simulink model "Offline_Preprocessing_ECGandSCG3D"  (R2019a)
settings: Solver=FixedStepDiscrete  StartTime=0.0  StopTime=param_sim_time  FixedStep=1/fs  MaxStep=1/fs  RelTol=1e-3
undefined symbols (not defined in the file): fdesignblkfcn, fs, gcbh
(part 1 of 3)
settings Model: PacingRate=100  Creator=rcord  LastModifiedBy=rcord
settings SolverCC: ZeroCrossControl=DisableAll
settings DataIOCC: ExternalInput=[t, signals.ecg.input, signals.scg.input_xyz]  LoadExternalInput=on  SignalLogging=off  DSMLogging=off  SaveTime=off  ReturnWorkspaceOutputs=off  TimeSaveName=t_preprocessing  OutputSaveName=out_preprocessing  LoggingIntervals=[-inf,inf]

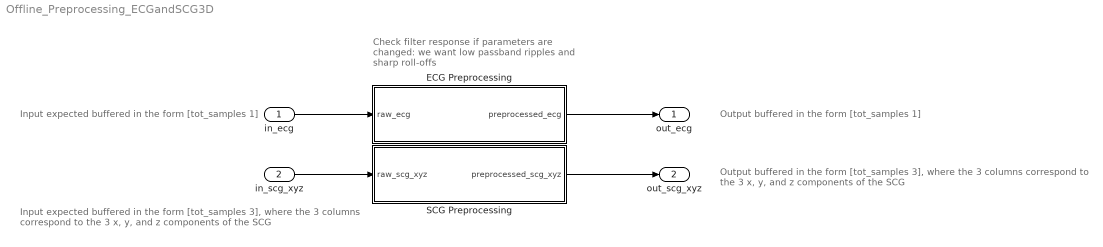
== system Offline_Preprocessing_ECGandSCG3D ==
  note: Input expected buffered in the form [tot_samples 3],
      | where the 3 columns correspond to the 3 x, y, and z components of the SCG
  note: Input expected buffered in the form [tot_samples 1]
  note: Check filter response if parameters are changed:
      | we want low passband ripples and sharp roll-offs
  note: Output buffered in the form [tot_samples 1]
  note: Output buffered in the form [tot_samples 3],
      | where the 3 columns correspond to the 3 x, y, and z components of the SCG
  in_ecg : Inport  SampleTime=1/fs
  in_scg_xyz : Inport  Port=2  SampleTime=1/fs
  ECG Preprocessing : Subsystem  mask{param_ecg_gain_mv=1000, param_ecg_fc_lo=2.05, param_ecg_fc_hi=36, param_ecg_trans_bw=2}
      mask prompts: param_ecg_gain_mv "mV Conversion Gain"; param_ecg_fc_lo "Low Passband Frequency Corner (Hz)"; param_ecg_fc_hi "High Passband Frequency Corner (Hz)"; param_ecg_trans_bw "Transition Bandwidth (Hz)"
      mask init:
      | assignin('base','param_ecg_gain_mv',param_ecg_gain_mv)
      | assignin('base','param_ecg_fc_lo',param_ecg_fc_lo)
      | assignin('base','param_ecg_fc_hi',param_ecg_fc_hi)
      | assignin('base','param_ecg_trans_bw',param_ecg_trans_bw)
      mask DialogControl DescGroupVar Prompt: ECG Preprocessing
      mask DialogControl DescTextVar Prompt: Preprocessing stage of the ECG. This involves conversion from V to mV and a filtfilt operation (i.e. a zero-phase FIR filtering) specified by the passband cornerns and transition bandwidth.
  SCG Preprocessing : Subsystem  mask{param_scg_gain_mg=3333, param_scg_fc_lo=7.5, param_scg_fc_hi=40, param_scg_trans_bw=2.5}
      mask prompts: param_scg_gain_mg "V to mg Conversion Gain"; param_scg_fc_lo "Low Passband Frequency Corner (Hz)"; param_scg_fc_hi "High Passband Frequency Corner (Hz)"; param_scg_trans_bw "Transition bandwidth"
      mask init:
      | assignin('base','param_scg_gain_mg',param_scg_gain_mg)
      | assignin('base','param_scg_fc_lo',param_scg_fc_lo)
      | assignin('base','param_scg_fc_hi',param_scg_fc_hi)
      | assignin('base','param_scg_trans_bw',param_scg_trans_bw)
      mask DialogControl DescGroupVar Prompt: SCG Preprocessing
      mask DialogControl DescTextVar Prompt: The SCG (x, y, and z) preprocessing block. This involves a V to mg conversion (determined by the transducer sensitivity) and a filtfilt operation. This filtfilt operation consists of a zero-phase FIR front-back filtering that is identical for each of the three cartesian acceleration components and is specified by the passband frequency corners and the transition bandwidth.
  out_ecg : Outport
  out_scg_xyz : Outport  Port=2
  wires:
  SCG Preprocessing/1(preprocessed_scg_xyz) -> out_scg_xyz/1
  ECG Preprocessing/1(preprocessed_ecg) -> out_ecg/1
  in_ecg/1 -> ECG Preprocessing/1(raw_ecg)
  in_scg_xyz/1 -> SCG Preprocessing/1(raw_scg_xyz)

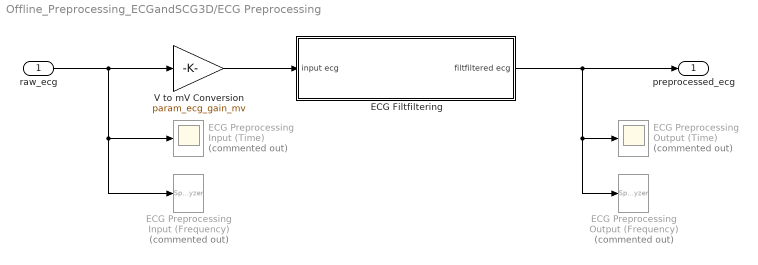
== system Offline_Preprocessing_ECGandSCG3D/ECG Preprocessing ==
  raw_ecg : Inport
  ECG Filtfiltering : Subsystem
  ECG Preprocessing Input (Frequency) : SpectrumAnalyzer  Commented=on
  ECG Preprocessing Input (Time) : Scope  Commented=on
  ECG Preprocessing Output (Frequency) : SpectrumAnalyzer  Commented=on
  ECG Preprocessing Output (Time) : Scope  Commented=on
  V to mV Conversion : Gain  Gain=param_ecg_gain_mv
  preprocessed_ecg : Outport
  wires:
  ECG Filtfiltering/1(filtfiltered ecg) -> preprocessed_ecg/1, ECG Preprocessing Output (Frequency)/1, ECG Preprocessing Output (Time)/1
  raw_ecg/1 -> V to mV Conversion/1, ECG Preprocessing Input (Frequency)/1, ECG Preprocessing Input (Time)/1
  V to mV Conversion/1 -> ECG Filtfiltering/1(input ecg)

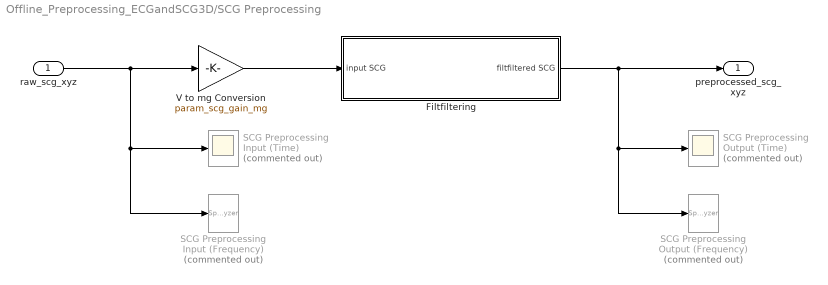
== system Offline_Preprocessing_ECGandSCG3D/SCG Preprocessing ==
  raw_scg_xyz : Inport
  Filtfiltering : Subsystem
  SCG Preprocessing Input (Frequency) : SpectrumAnalyzer  Commented=on
  SCG Preprocessing Input (Time) : Scope  Commented=on
  SCG Preprocessing Output (Frequency) : SpectrumAnalyzer  Commented=on
  SCG Preprocessing Output (Time) : Scope  Commented=on
  V to mg Conversion : Gain  Gain=param_scg_gain_mg
  preprocessed_scg_xyz : Outport
  wires:
  V to mg Conversion/1 -> Filtfiltering/1(" input SCG")
  Filtfiltering/1(filtfiltered SCG) -> preprocessed_scg_xyz/1, SCG Preprocessing Output (Frequency)/1, SCG Preprocessing Output (Time)/1
  raw_scg_xyz/1 -> V to mg Conversion/1, SCG Preprocessing Input (Frequency)/1, SCG Preprocessing Input (Time)/1

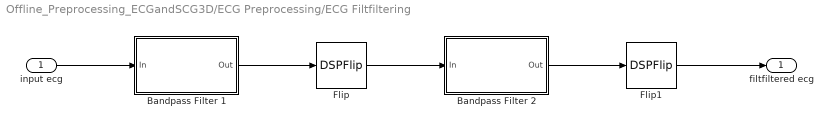
== system Offline_Preprocessing_ECGandSCG3D/ECG Preprocessing/ECG Filtfiltering ==
  input ecg : Inport
  Bandpass Filter 1 : Subsystem  DialogController=fdesignblkfcn  InitFcn=fdesignblkfcn(gcbh, {'InitFcn'});  mask(Bandpass Filter){}
      mask help: Design a bandpass filter
      settings: CopyFcn=fdesignblkfcn(gcbh, {'CopyFcn'});
      mask Help: helpview(mapfilelocation('dsp'), 'dspbandpassfilter');
      mask Display: disp('Bandpass');
  Bandpass Filter 2 : Subsystem  DialogController=fdesignblkfcn  InitFcn=fdesignblkfcn(gcbh, {'InitFcn'});  mask(Bandpass Filter){}
      mask help: Design a bandpass filter
      settings: CopyFcn=fdesignblkfcn(gcbh, {'CopyFcn'});
      mask Help: helpview(mapfilelocation('dsp'), 'dspbandpassfilter');
      mask Display: disp('Bandpass');
  Flip : DSPFlip
  Flip1 : DSPFlip
  filtfiltered ecg : Outport
  wires:
  Flip/1 -> Bandpass Filter 2/1(In)
  input ecg/1 -> Bandpass Filter 1/1(In)
  Flip1/1 -> filtfiltered ecg/1
  Bandpass Filter 1/1(Out) -> Flip/1
  Bandpass Filter 2/1(Out) -> Flip1/1

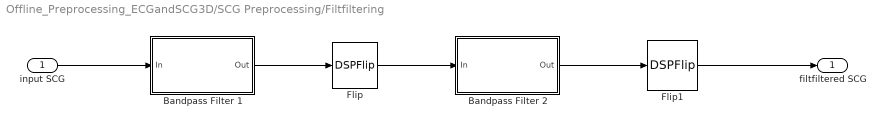
== system Offline_Preprocessing_ECGandSCG3D/SCG Preprocessing/Filtfiltering ==
  " input SCG" : Inport
  Bandpass Filter 1 : Subsystem  DialogController=fdesignblkfcn  InitFcn=fdesignblkfcn(gcbh, {'InitFcn'});  mask(Bandpass Filter){}
      mask help: Design a bandpass filter
      settings: CopyFcn=fdesignblkfcn(gcbh, {'CopyFcn'});
      mask Help: helpview(mapfilelocation('dsp'), 'dspbandpassfilter');
      mask Display: disp('Bandpass');
  Bandpass Filter 2 : Subsystem  DialogController=fdesignblkfcn  InitFcn=fdesignblkfcn(gcbh, {'InitFcn'});  mask(Bandpass Filter){}
      mask help: Design a bandpass filter
      settings: CopyFcn=fdesignblkfcn(gcbh, {'CopyFcn'});
      mask Help: helpview(mapfilelocation('dsp'), 'dspbandpassfilter');
      mask Display: disp('Bandpass');
  Flip : DSPFlip
  Flip1 : DSPFlip
  filtfiltered SCG : Outport
  wires:
  Bandpass Filter 2/1(Out) -> Flip1/1
  Bandpass Filter 1/1(Out) -> Flip/1
  Flip1/1 -> filtfiltered SCG/1
  " input SCG"/1 -> Bandpass Filter 1/1(In)
  Flip/1 -> Bandpass Filter 2/1(In)

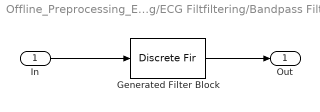
== system Offline_Preprocessing_ECGandSCG3D/ECG Preprocessing/ECG Filtfiltering/Bandpass Filter 1 ==
  In : Inport
  Generated Filter Block : DiscreteFir  Tag=BlockMethodSubSystem  Coefficients=[-0.0116406344063622168 0.00576809638741981705 0.00412102174232116189 0.00269274783173200846 0.00147079622405396279 0.000491631581443595714 -0.000279527338118035207 -0.000824440163218089286 -0.0011931089442172027 -0.00137786624889967881 -0.00143680610402490035 -0.0013658599370285178 -0.00122537593751419899 -0.00100892957375263437 -0.000775151304297802199 -0.000510774577038271629 -0.00027121264178328261 -3.21617788413223332e-05 0.000150365289888468659 0.000323517566100257545 0.000410189273670719806 0.00049803134316846881 0.000505564927906845124 0.000475157220458219745 0.000425303838401711043 0.000342667518480603561 0.000218386639681151032 9.32202317054566659e-05 -3.87356123631495824e-05 -0.000159506396561761091 -0.00028910293766154678 -0.000397731647781897693 -0.0004962822578398942 -0.000556158228593433418 -0.000601142291741041737 -0.00061032042524469636 -0.000610411153005745166 -0.000575325879602293574 -0.000532487836056453126 -0.000454667284566329447 -0.000377559062145994481 -0.000278724916437145948 -0.000187745128628987248 -9.74324644924737249e-05 -1.60738650468866817e-05 5.9764814736124397e-05 0.000109987183421211138 0.000157422257216391359 0.000176177967607079114 0.00018056911694317411 0.000152238854462556986 0.000116164138403226577 5.20308008613596523e-05 -1.73239994344202841e-05 -0.000108419462697777885 -0.000192758346105910763 -0.000288114649125117278 -0.00036987488099304508 -0.00045763639443521624 -0.000524326642655037131 -0.00058632464066331845 -0.000620766605119459774 -0.00064268165693386059 -0.000638078579740596064 -0.000620092611563771018 -0.000572834914300220099 -0.000519984983498502501 -0.000440578049522327708 -0.000362776463167686913 -0.000271958458209525106 -0.000191413582727147438 -0.000103296930882701768 -3.48626201441531308e-05 3.13573430135057063e-05 7.15775158072421563e-05 0.000103833267199419932 0.000103391792586697215 9.08011246543508066e-05 4.6939312636908731e-05 -5.62656538495055758e-06 -8.48056019403329447e-05 -0.000169065203230319219 -0.000271297028825072742 -0.000368012740422246978 -0.00047280159332896074 -0.000559355242459418089 -0.000646838198869518349 -0.000706291730566098452 -0.000756959227202433707 -0.000776213928397353342 -0.00078351986501341668 -0.000757139075089350091 -0.000720571226219025862 -0.000653100073902892694 -0.000578446102546691446 -0.000480516490167021831 -0.000386704679715342906 -0.000280864569862355681 -0.000188982750800533589 -9.63843912055121349e-05 -2.87701546104728728e-05 2.98969073572342287e-05 5.62378466815432326e-05 6.85710121285463409e-05 4.34826849005191807e-05 5.4043371536319218e-06 -6.74672227912870293e-05 -0.000148541085202819056 -0.000256137309555011863 -0.000364360021022150371 -0.000487775998109139797 -0.000597948333952508931 -0.000711693120677205429 -0.000801648264494816964 -0.000884116668799860006 -0.000934017261241329444 -0.000969583957585701262 -0.000967017051073068221 -0.000947278381884976081 -0.000890870622043564431 -0.000821286176068025675 -0.000720694584109535935 -0.000616440121337090766 -0.000492831386257134782 -0.000379545392445496468 -0.000259339184515096702 -0.00016178941864374366 -7.10042565194822506e-05 -1.3392901324712006e-05 2.78153978735731083e-05 2.90754142912783009e-05 1.10946459254170071e-05 -4.76087551916030277e-05 -0.000122756950540332116 -0.000231389766655416482 -0.000347967152363855281 -0.00048791369964742981 -0.000622520837549468686 -0.000765575302446700606 -0.000888640186329310924 -0.00100616465864617095 -0.00109050986367765362 -0.00115914378470589191 -0.00118627235524722263 -0.00119192917236833271 -0.00115382032932690066 -0.00109540150637619203 -0.000999331912807106815 -0.000890174731215546966 -0.000753722389353950195 -0.000618155844393425413 -0.000470259752504975648 -0.000339360741956546905 -0.000212343108328122768 -0.000116871493706854207 -3.89508706146440148e-05 -3.8656480634054885e-06 6.81299165694246311e-06 -2.87912369563211173e-05 -8.92169780942544954e-05 -0.000192214698281994306 -0.000312039737549282131 -0.000463894441742667904 ...(+18228 chars)]  InputProcessing=Columns as channels (frame based)
  Out : Outport
  wires:
  In/1 -> Generated Filter Block/1
  Generated Filter Block/1 -> Out/1
